simulink model "mech_spen"  (Simulink 7.1)
settings: Solver=ode45  StartTime=0.0  StopTime=inf  RelTol=1e-5  AbsTol=1e-8
libraries: mblibv1 x5, simulink x1
Description:
  | Simple Pendulum
  | 
  | A rod swinging in gravity by one revolute joint. Scope shows angle and angular velocity. XY Graph shows model phase space.
settings Model: Creator=arnav  LastModifiedBy=Administrator  ExtModeAutoUpdateStatusClock=off
settings DataIOCC: SignalLoggingName=sigsOut
settings OptimizationCC: BooleanDataType=off  InlineInvariantSignals=on
settings DebuggingCC: SaveWithParameterizedLinksMsg=none  CheckExecutionContextPreStartOutputMsg=on  CheckExecutionContextRuntimeOutputMsg=on  SignalResolutionControl=TryResolveAllWithWarning  SolverPrmCheckMsg=none  MultiTaskDSMMsg=warning  MultiTaskCondExecSysMsg=none  SigSpecEnsureSampleTimeMsg=none  StrictBusMsg=None
settings HardwareCC: TargetEndianess=LittleEndian  TargetHWDeviceType=MATLAB Host  ProdEqTarget=off
settings RTWCC: SystemTargetFile=rsim.tlc  TemplateMakefile=rsim_default_tmf  Description=Rapid Simulation Target  ProcessScript=rsim_make_rtw_hook  IncludeERTFirstTime=on
settings RSimTargetCC: TargetFcnLib=ansi_tfl_tmw.mat  TargetFunctionLibrary=ANSI_C  IsPILTarget=off  EnableShiftOperators=on  PortableWordSizes=off

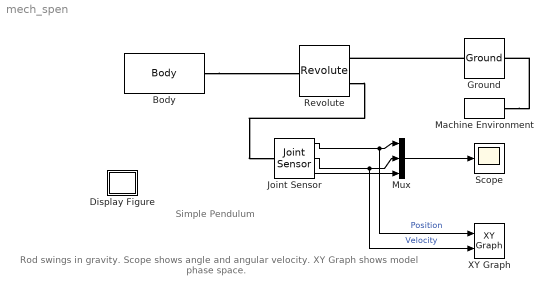
== system mech_spen ==
  note: Rod swings in gravity. Scope
      | shows angle and angular velocity.
      | XY Graph shows model phase space.
  note: Simple Pendulum
  Body : mblibv1/Bodies/Body  Orientation=left  DialogController=MECH.DynMechDlgSource  PhysicalDomain=mechanical  SubClassName=Unknown  LeftPortType=workingframe  RightPortType=workingframe  LConnTagsString=CS1  DialogClass=MechanicalBodyBlock  Mass=2490  MassUnits=g  InertiaUnits=kg*m^2  Inertia=[ 1.25e-4 0 0; 0 0.83 0; 0 0 0.83]  Shape=Cylinder  ShapeDims=[1 1]  ShapeUnits=m  ShapeUse=false  Density=1  DensityUnits=kg/m^3  DensityUse=false  GraphicsMode=1  BodyColor=[0.5 0.5 0.5]  GraphicsObj=[]  AttachedToCS=1  CG=Left$CG$[3.01745 3.5003 5]$WORLD$WORLD$m$[0 0 0]$Euler X-Y-Z$deg$WORLD$false$none  WorkingFrames=Left$CS1$[3 4 5]$WORLD$WORLD$m$[0 0 0]$Euler X-Y-Z$deg$WORLD$true$none  CGPos=[3.01745 3.5003 5]  CGRot=[0 0 0]  CS0Pos=[]  CS0Rot=[]  CS1Pos=[3 4 5]  CS1Rot=[0 0 0]  CS2Pos=[]  CS2Rot=[]  CS3Pos=[]  CS3Rot=[]  CS4Pos=[]  CS4Rot=[]  CS5Pos=[]  CS5Rot=[]  CS6Pos=[]  CS6Rot=[]  CS7Pos=[]  CS7Rot=[]  CS8Pos=[]  CS8Rot=[]  CS9Pos=[]  CS9Rot=[]  CS10Pos=[]  CS10Rot=[]  CS11Pos=[]  CS11Rot=[]  CS12Pos=[]  CS12Rot=[]  CS13Pos=[]  CS13Rot=[]  CS14Pos=[]  CS14Rot=[]  CS15Pos=[]  CS15Rot=[]  CS16Pos=[]  CS16Rot=[]  CS17Pos=[]  CS17Rot=[]  CS18Pos=[]  CS18Rot=[]  CS19Pos=[]  CS19Rot=[]  CS20Pos=[]  CS20Rot=[]
  Display Figure : Subsystem  Description="Help callback for simple pendulum model: mech_spen.mdl.  Opens Help browser to Type 19 marker at documentation for this tutorial model."
      settings: OpenFcn=helpview([docroot '/toolbox/physmod/mech/mech.map'], 'mech_spen_help');
      mask Type: Help callback
      mask Display: image(imread('info.bmp'))
  Ground : mblibv1/Bodies/Ground  Orientation=left  DialogController=MECH.DynMechDlgSource  SystemSampleTime=-1  LeftPortType=env  RightPortType=workingframe  PhysicalDomain=Mechanical  DialogClass=GroundBlock  CoordPosition=[3 4 5]  CoordPositionUnits=m  StateVectorMgrId=1  MachineId=[2 0]  ShowEnvPort=on
  Joint Sensor : mblibv1/Sensors &  Actuators/Joint Sensor  DialogController=MECH.DynMechDlgSource  SystemSampleTime=-1  PhysicalDomain=Mechanical  PortType=blob  Muxed=off  Pose=off  Angle=on  AngleUnits=deg  ArcVelocity=on  ArcVelocityUnits=deg/s  ArcAcceleration=off  ArcAccelerationUnits=deg/s^2  CoordPosition=on  CoordPositionUnits=m  Velocity=off  VelocityUnits=m/s  Acceleration=off  AccelerationUnits=m/s^2  Quaternion=on  QuaternionDT=off  QuaternionDDT=off  QuaternionUnits=off  OutputVector=[ 1 1 ]  ActiveIO=on  Width=5  DialogClass=MechanicalSensorBlock  Primitive=R1  Force=off  ForceUnits=N  Torque=off  TorqueUnits=N*m  ReferenceFrame=Absolute (INERTIAL)  ReactionSensedSide=Base  ReactionReferenceFrame=Absolute (World)  ReactionForce=on  ReactionForceUnits=N  ReactionMoment=off  ReactionMomentUnits=N*m
  Machine Environment : mblibv1/Bodies/Machine Environment  Tag=Factory ground  DialogController=MECH.DialogSource  SystemSampleTime=-1  PortType=env  PhysicalDomain=Mechanical  DialogTemplateClass=MECH.MachineEnvironment  SyncWhenCopied=off  Gravity=[0 -9.81 0]  GravityUnits=m/s^2  GravityAsSignal=off  Dimensionality=3D Only  AnalysisType=Forward dynamics  LinearAssemblyTolerance=1e-3  LinearAssemblyToleranceUnits=m  AngularAssemblyTolerance=1e-3  AngularAssemblyToleranceUnits=rad  ConstraintSolverType=Stabilizing  ConstraintRelTolerance=1e-4  ConstraintAbsTolerance=1e-4  UseRobustSingularityHandling=off  RedundancyAnalysisToleranceType=Automatically select tolerance  RedundancyAnalysisTolerance=1e-14  StatePerturbationType=Fixed  PerturbationSize=1e-5  VisualizeMachine=on
  Mux : Mux  Inputs=3
  Revolute : mblibv1/Joints/Revolute  Orientation=left  DialogController=MECH.DynMechDlgSource  PhysicalDomain=mechanical  SubClassName=Unknown  LeftPortType=blob  RightPortType=blob  LConnTagsString=__newl0|SA1  RConnTagsString=__newr0  NumSAPorts=1  CutJoint=off  MarkAsCut=off  Primitives=revolute  PrimitiveProps=R1$WORLD$[0 0 1]$revolute  DialogClass=JointBlock  R1Axis=[0 0 1]
  Scope : Scope
      settings: YMin=-225  YMax=150
  XY Graph : simulink/Sinks/XY Graph  SystemSampleTime=-1  xmin=-25  xmax=200  ymin=-500  ymax=500  st=-1
  wires:
  Joint Sensor/1 -> Mux/1, XY Graph/1  "Position"
  Joint Sensor/2 -> Mux/2, XY Graph/2  "Velocity"
  Mux/1 -> Scope/1
  Joint Sensor/3 -> Mux/3
  connections:
  Ground/RConn1 -- Revolute/LConn1
  Revolute/LConn2 -- Joint Sensor/LConn1
  Body/LConn1 -- Revolute/RConn1
  Machine Environment/RConn1 -- Ground/LConn1

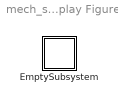
== system mech_spen/Display Figure ==
  EmptySubsystem : Subsystem

== system mech_spen/Display Figure/EmptySubsystem ==
